simulink library "init"  (R2024a)
settings: Solver=VariableStepAuto  StartTime=0.0  StopTime=10.0  RelTol=1e-3
settings Model: Creator=adriaeik  LastModifiedBy=adriaeik

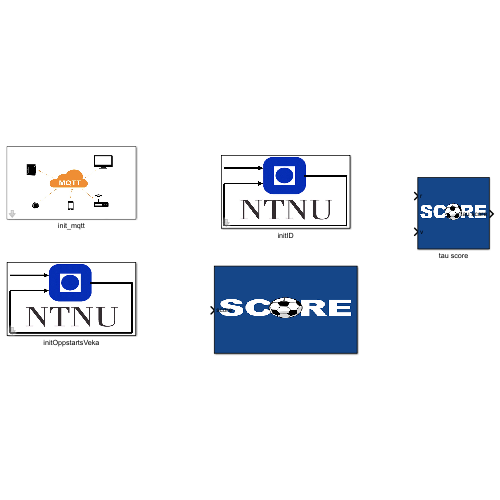
[thumbnail: Simulink's stored preview of the top-level diagram]
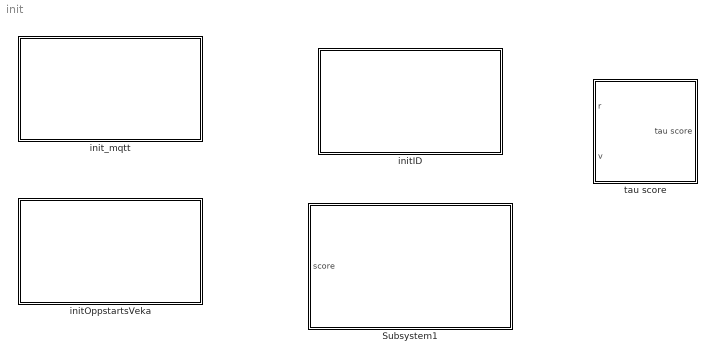
== system init ==
  Subsystem1 : Subsystem
      mask Display: image('score.png');
  initID : Subsystem  mask{carID=0, groupID=0}
      mask prompts: carID "Zumo Car ID"; groupID "Group ID"
      mask Display: image('kyb.png');
  initOppstartsVeka : Subsystem  mask{carID=14, groupID=14}
      mask prompts: carID "Zumo Car ID"; groupID "Group ID"
      mask Display: image('pic/kyb.png');
  init_mqtt : Subsystem  mask{carID=14, groupID=14, brokerVal='192.168.1.3', portVal='1883', userVal='BIAISbroker', passVal='shinyteapot294'}
      mask prompts: carID "Zumo Car ID"; groupID "Group ID"; brokerVal "Broker"; portVal "MQTT-port"; userVal "Username"; passVal "Password"
      mask Display: image('pic/mqtt.png');
  tau score : Subsystem
      mask Display: image('score.png');

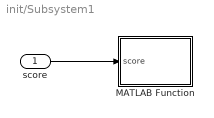
== system init/Subsystem1 ==
  score : Inport
  MATLAB Function : MATLAB Function  TreatAsAtomicUnit=on
  wires:
  score/1 -> MATLAB Function/1(score)

== system init/initID ==

== system init/initOppstartsVeka ==

== system init/init_mqtt ==

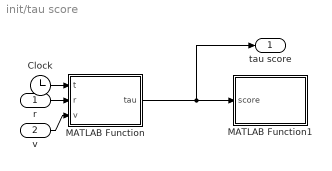
== system init/tau score ==
  r : Inport
  v : Inport  Port=2
  Clock : Clock
  MATLAB Function : MATLAB Function  TreatAsAtomicUnit=on
  MATLAB Function1 : MATLAB Function  TreatAsAtomicUnit=on
  tau score : Outport
  wires:
  MATLAB Function/1(tau) -> tau score/1, MATLAB Function1/1(score)
  Clock/1 -> MATLAB Function/1(t)
  v/1 -> MATLAB Function/3(v)
  r/1 -> MATLAB Function/2(r)

== matlab function init/tau score/MATLAB Function ==
  settings: updateMethod=DISCRETE
  data: t input; r input; tau output; v input
function tau = fcn(t, r, v)
    persistent tau_val tolerance overshoot_detected prev_v prev_t settled_count
    
    % Initialize persistent variables
    if isempty(tau_val)
        tau_val = inf;
        tolerance = 0.01 * r;  % 1% tolerance
        overshoot_detected = false;
        prev_v = v;
        prev_t = t;
        settled_count = 0;
    end
    
    % Check if velocity has reached 63.2% of reference (time constant point)
    reference_63_percent = r * (1 - exp(-1));
    
    % Only set tau ONCE when velocity first reaches this reference point
    if isinf(tau_val) && (v >= reference_63_percent) && ~overshoot_detected
        tau_val = t;  % Lock it in
        % Debug: uncomment to see when this happens
        % fprintf('TAU SET TO: %.3f at time %.3f\n', tau_val, t);
    end
    
    % Check for excessive overshoot - this might be causing the reset
    if v > r + tolerance
        if ~overshoot_detected  % Only print once
            % fprintf('OVERSHOOT DETECTED at t=%.3f, v=%.3f > r+tol=%.3f\n', t, v, r+tolerance);
        end
        overshoot_detected = true;
        tau_val = inf;  % This resets tau!
    end
    
    % Steady-state error detection
    dt = t - prev_t;
    if dt > 0.01
        velocity_change = abs(v - prev_v);
        steady_state_error = abs(v - r) > tolerance;
        velocity_settled = velocity_change < 0.001;
        
        if steady_state_error && velocity_settled
            settled_count = settled_count + 1;
            if settled_count > 500  % Increase from 200 to 500 (5 seconds instead of 2)
                tau_val = inf;
            end
        else
            settled_count = 0;
        end
        
        prev_v = v;
        prev_t = t;
    end
    
    tau = tau_val;
end

== matlab function init/Subsystem1/MATLAB Function ==
  data: score input
function fcn(score)
 assignin('base', 'score', score);

== matlab function init/tau score/MATLAB Function1 ==
  data: score input
function fcn(score)
if score == inf
    score = 9999999;
end
 assignin('base', 'score', score);
